simulink model "khaosatthoigian"  (R2022a)
settings: Solver=FixedStepAuto  StartTime=0.0  StopTime=20  RelTol=1e-3
libraries: arduinolib x2
settings Model: ExtModeTrigDuration=2  Creator=TUAN  LastModifiedBy=TUAN
settings OptimizationCC: EnhancedBackFolding=on  PassReuseOutputArgsAs=Individual arguments  ZeroExternalMemoryAtStartup=off  ZeroInternalMemoryAtStartup=off  MaxStackSize=64  OptimizeBlockOrder=speed  DifferentSizesBufferReuse=on  OptimizationCustomize=off  EfficientTunableParamExpr=on
settings DebuggingCC: ParameterTunabilityLossMsg=error
settings HardwareCC: ProdBitPerPointer=32  ProdBitPerSizeT=32  ProdBitPerPtrDiffT=32  ProdLargestAtomicInteger=Long  ProdLargestAtomicFloat=Double  ProdWordSize=32  ProdHWDeviceType=ARM Compatible->ARM Cortex
settings SFSimCC: MATLABDynamicMemAlloc=off
settings RTWCC: SystemTargetFile=ert.tlc  HardwareBoard=ESP32-WROOM(Arduino Compatible)  TLCOptions="-aInlineSetEventsForThisBaseRateFcn=TLC_FALSE -aSuppressMultiTaskScheduler=TLC_FALSE  -aRateBasedStepFcn=0"  TemplateMakefile=ert_default_tmf  Toolchain=ESP32
settings CodeAppCC: ForceParamTrailComments=on  IgnoreCustomStorageClasses=off  OperatorAnnotations=on  SimulinkDataObjDesc=on  SFDataObjDesc=on  InsertBlockDesc=on
settings ERTTargetCC: SupportContinuousTime=on  SupportVariableSizeSignals=on  ExtModeTransport=3  ExtModeStaticAlloc=on  ExtModeStaticAllocSize=65536  ExtModeMexFile=ext_xcp  ExtModeIntrfLevel=Level2 - Open

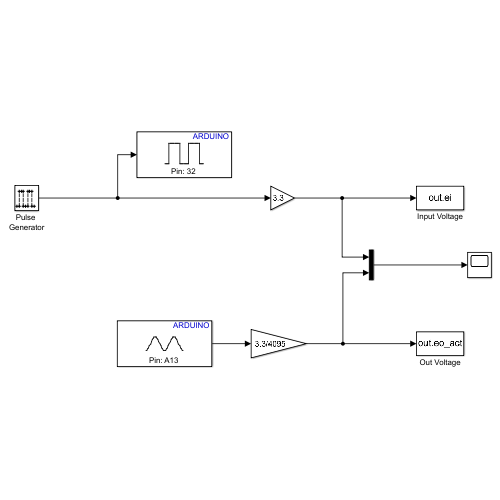
[thumbnail: Simulink's stored preview of the top-level diagram]
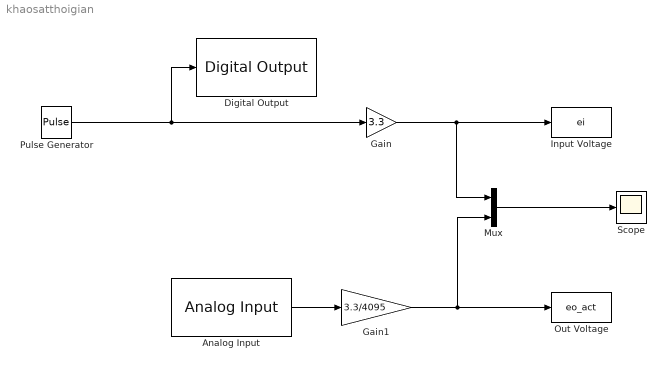
== system khaosatthoigian ==
  Analog Input : arduinolib/Analog Input  pinNumber=13  ReadResultsOnly=off  ConversionTriggerSource=Software  ExternalTriggerType=uint32( 0 )  OutputDataType=uint16  EnableConversionCompleteNotify=off  EnableOuputStatus=off  SampleTime=0.1  blockPlatform=arduino
  Digital Output : arduinolib/Digital Output  pinNumber=32  Direction=output  blockPlatform=arduino
  Gain : Gain  Gain=3.3
  Gain1 : Gain  Gain=3.3/4095  OutDataTypeStr=double
  Input Voltage : ToWorkspace  VariableName=ei  SampleTime=-1
  Mux : Mux  Inputs=2
  Out Voltage : ToWorkspace  VariableName=eo_act  SampleTime=-1
      settings: Save2DSignal=2-D array (concatenate along first dimension)
  Pulse Generator : DiscretePulseGenerator  Period=100  PulseWidth=50  SampleTime=0.1
  Scope : Scope
  wires:
  Gain1/1 -> Mux/2, Out Voltage/1
  Mux/1 -> Scope/1
  Gain/1 -> Mux/1, Input Voltage/1
  Pulse Generator/1 -> Digital Output/1, Gain/1
  Analog Input/1 -> Gain1/1
